simulink model "PIL_lqr_lin"  (R2024b)
settings: Solver=VariableStepAuto  StartTime=0.0  StopTime=params.simtime  RelTol=1e-3
values from neighbouring files (symbols this model uses):
  params = parameters()    [lqr_STM_compare.m]    (also in lqr_compare.m; lqr_main_isolated.m)
  s = serialport('/dev/cu.usbmodem21103', 921600, 'Timeout', 0.25)    [lqr_STM_compare.m]
undefined symbols (not defined in the file or in its folder): controller_stm, nl_model
settings Model: Creator=ben83  LastModifiedBy=ben
settings RTWCC: GPUComputeCapability=3.5

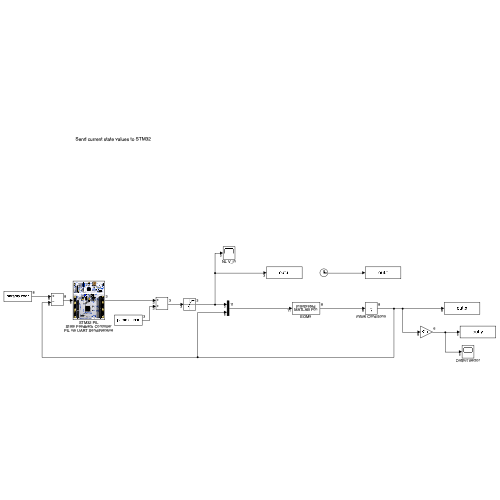
[thumbnail: Simulink's stored preview of the top-level diagram]
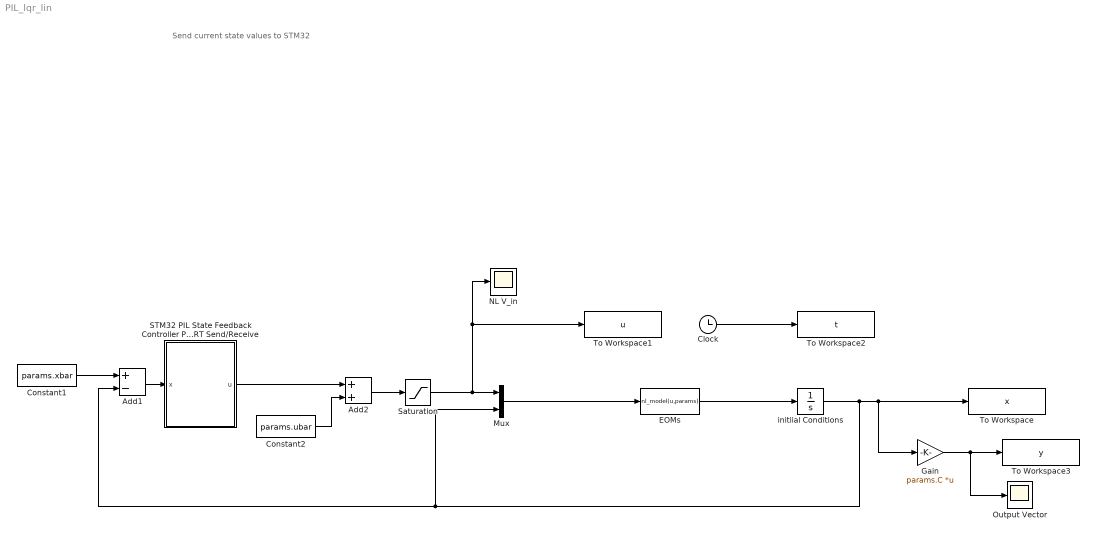
== system PIL_lqr_lin ==
  note: Send current state values to STM32
  Add1 : Sum  Inputs=+-
  Add2 : Sum
  Clock : Clock
  Constant1 : Constant  Value=params.xbar
  Constant2 : Constant  Value=params.ubar
  EOMs : MATLABFcn  MATLABFcn=nl_model(u,params)  OutputDimensions=8
  Gain : Gain  Gain=params.C  Multiplication=Matrix(K*u)
  Mux : Mux  Inputs=2
  NL V_in : Scope
  Output Vector : Scope
  STM32 PIL State Feedback Controller PIL via UART Send/Receive : Subsystem
      mask Display: image('$imagefile'); % Use "Edit Image" on toolstrip to change.
  Saturation : Saturate  UpperLimit=10.8  LowerLimit=-10.8
  To Workspace : ToWorkspace  VariableName=x  SampleTime=-1
  To Workspace1 : ToWorkspace  VariableName=u  SampleTime=-1
  To Workspace2 : ToWorkspace  VariableName=t  SampleTime=-1
  To Workspace3 : ToWorkspace  VariableName=y  SampleTime=-1
  initiial Conditions : Integrator  InitialCondition=params.ic
  wires:
  EOMs/1 -> initiial Conditions/1
  Mux/1 -> EOMs/1
  Clock/1 -> To Workspace2/1
  Add2/1 -> Saturation/1
  initiial Conditions/1 -> Add1/2, Mux/2, Gain/1, To Workspace/1
  Gain/1 -> Output Vector/1, To Workspace3/1
  Constant1/1 -> Add1/1
  Constant2/1 -> Add2/2
  STM32 PIL State Feedback Controller PIL via UART Send/Receive/1(u) -> Add2/1
  Add1/1 -> STM32 PIL State Feedback Controller PIL via UART Send/Receive/1(x)
  Saturation/1 -> NL V_in/1, To Workspace1/1, Mux/1

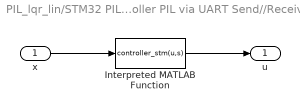
== system PIL_lqr_lin/STM32 PIL State Feedback Controller PIL via UART Send//Receive ==
  x : Inport
  Interpreted MATLAB Function : MATLABFcn  MATLABFcn=controller_stm(u,s)
  u : Outport
  wires:
  x/1 -> Interpreted MATLAB Function/1
  Interpreted MATLAB Function/1 -> u/1
